simulink model "ex4_sim"  (R2015b)
settings: Solver=VariableStepAuto  StartTime=0.0  StopTime=simtime  RelTol=1e-3
values from neighbouring files (symbols this model uses):
  enable_karnop = 1    [ex1.m]    (also in ex2.m = 0; ex3.m; ex4.m = 0; exall.m = 0)
  enable_sin = 1    [ex1.m]    (also in ex2.m = 0; ex3.m; ex4.m = 0; exall.m = 0)
  F_c = 0.001    [ex1.m]    (also in ex2.m; ex3.m; ex4.m; exall.m)
  J = (J1 + J2)    (= 3.6e-05)    [ex1.m]    (also in ex2.m; ex3.m; ex4.m)
  motor = motor_pars    [ex1.m]    (also in ex2.m; ex3.m; ex4.m)
  motor_L = motor_pars    [ex1.m]    (also in ex2.m; ex3.m; ex4.m)
  n = 5    [ex1.m]    (also in ex2.m; ex3.m; ex4.m; ex5.m)
  sim_step_v = 2.38    [ex1.m]    (also in ex2.m = 1; ex3.m; ex4.m = 10)
undefined symbols (not defined in the file or in its folder): T_fric
libraries: simulink x2
settings Model: Creator=gabras  LastModifiedBy=Lamn
settings SolverCC: ZeroCrossAlgorithm=Adaptive
settings DataIOCC: SaveFormat=Array
settings DebuggingCC: SolverPrmCheckMsg=warning
settings HardwareCC: ProdBitPerPointer=32  ProdLargestAtomicFloat=None  ProdIntDivRoundTo=Undefined  ProdEndianess=Unspecified  ProdWordSize=32  ProdHWDeviceType=32-bit Generic
settings GRTTargetCC: GeneratePreprocessorConditionals=Disable all
settings ConfigComp: CovModelRefEnable=Off  CovSFcnEnable=off

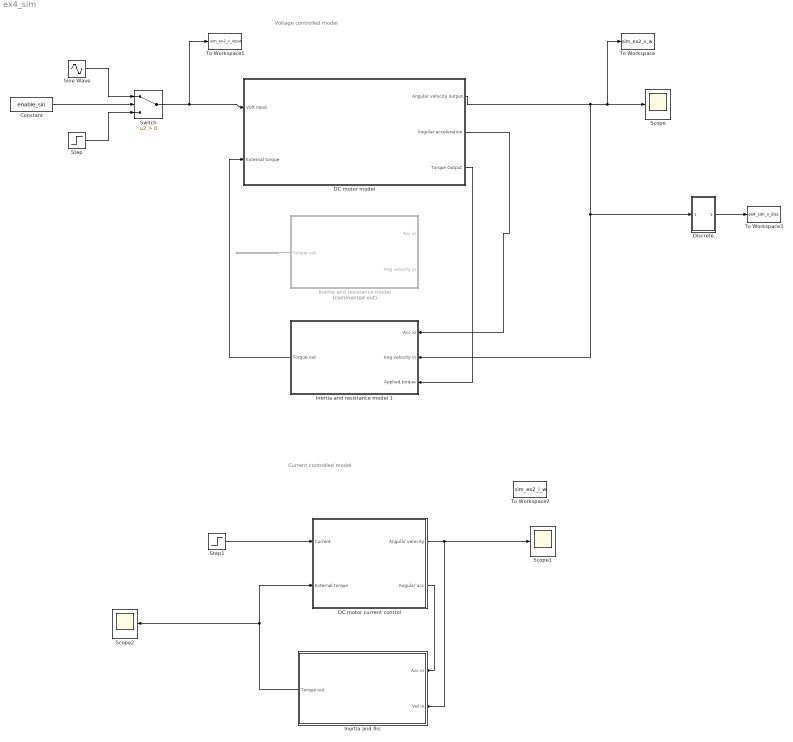
== system ex4_sim ==
  note: Current controlled model
  note: Voltage controlled model
  Constant : Constant  Value=enable_sin
  "DC motor current control " : Subsystem
  DC motor model : Subsystem
  Discrete : Subsystem
  Inertia and firc : Subsystem
  "Inertia and resistance model " : Subsystem  Commented=on
  Inertia and resistance model 1 : Subsystem
  Scope : Scope
  Scope1 : Scope
  Scope2 : Scope
  Sine Wave : Sin  SampleTime=0
  Step : Step  Time=0  After=sim_step_v  SampleTime=0
  Step1 : Step  Time=0  SampleTime=0
  Switch : Switch  Criteria=u2 > Threshold
  To Workspace : ToWorkspace  VariableName=sim_ex2_v_w  SaveFormat=Timeseries  SampleTime=-1
  To Workspace1 : ToWorkspace  VariableName=sim_ex2_v_input  SaveFormat=Timeseries  SampleTime=-1
  To Workspace2 : ToWorkspace  VariableName=sim_ex2_i_w  SaveFormat=Timeseries  SampleTime=-1
  To Workspace3 : ToWorkspace  VariableName=ex4_sim_v_disc  SaveFormat=Timeseries  SampleTime=-1
  wires:
  "Inertia and resistance model "/1(Torque out) -> ?
  DC motor model/2("Angular acceleration ") -> Inertia and resistance model 1/1(Acc in)
  Step1/1 -> "DC motor current control "/1(Current)
  "DC motor current control "/1(Angular velocity) -> Scope1/1, Inertia and firc/2(Vel in)
  "DC motor current control "/2(Angular acc) -> Inertia and firc/1(Acc in)
  Inertia and firc/1(Torque out) -> Scope2/1, "DC motor current control "/2(External torque)
  Step/1 -> Switch/3
  Sine Wave/1 -> Switch/1
  Switch/1 -> To Workspace1/1, DC motor model/1("Volt input ")
  Constant/1 -> Switch/2
  Inertia and resistance model 1/1(Torque out) -> DC motor model/2(External torque)
  DC motor model/3(Torque Output) -> Inertia and resistance model 1/3(Applied torque)
  DC motor model/1("Angular velocity output ") -> Discrete/1(In1), Inertia and resistance model 1/2(Ang velocity in), To Workspace/1, Scope/1
  Discrete/1(Out1) -> To Workspace3/1

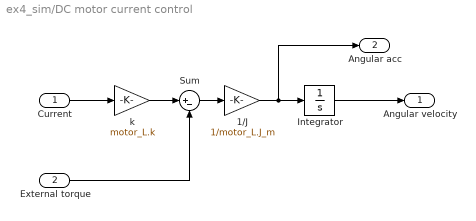
== system ex4_sim/DC motor current control  ==
  Current : Inport
  External torque : Inport  Port=2
  1/J : Gain  Gain=1/motor_L.J_m
  Integrator : Integrator
  Sum : Sum  Inputs=|+-
  "k " : Gain  Gain=motor_L.k
  Angular velocity : Outport
  Angular acc : Outport  Port=2
  wires:
  Current/1 -> "k "/1
  External torque/1 -> Sum/2
  "k "/1 -> Sum/1
  Sum/1 -> 1/J/1
  1/J/1 -> Angular acc/1, Integrator/1
  Integrator/1 -> Angular velocity/1

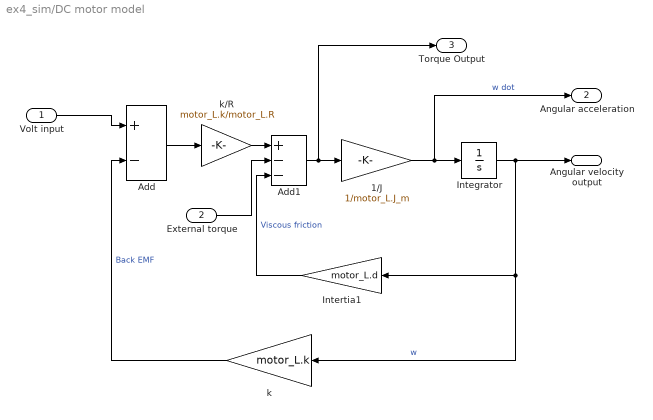
== system ex4_sim/DC motor model ==
  "Volt input " : Inport
  External torque : Inport  Port=2
  1/J : Gain  Gain=1/motor_L.J_m
  Add : Sum  Inputs=+-
  Add1 : Sum  Inputs=+--
  Integrator : Integrator
  Intertia1 : Gain  Gain=motor_L.d
  k : Gain  Gain=motor_L.k
  "k/R " : Gain  Gain=motor_L.k/motor_L.R
  "Angular velocity output " : Outport
  "Angular acceleration " : Outport  Port=2
  Torque Output : Outport  Port=3
  wires:
  "Volt input "/1 -> Add/1
  k/1 -> Add/2  "Back EMF"
  Add/1 -> "k/R "/1
  "k/R "/1 -> Add1/1
  Add1/1 -> Torque Output/1, 1/J/1
  1/J/1 -> "Angular acceleration "/1, Integrator/1  "w dot"
  Integrator/1 -> "Angular velocity output "/1, k/1, Intertia1/1  "w"
  External torque/1 -> Add1/2
  Intertia1/1 -> Add1/3  "Viscous friction"

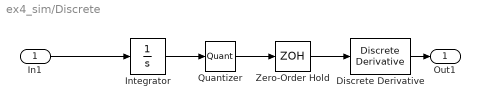
== system ex4_sim/Discrete ==
  In1 : Inport
  Discrete Derivative : simulink/Discrete/Discrete Derivative  gainval=1.0  ICPrevScaledInput=0.0  InputProcessing=Inherited  OutMin=[]  OutMax=[]  OutDataType=fixdt(1, 16)  OutScaling=2^-10  DoSatur=off
  Integrator : Integrator
  Quantizer : Quantizer  QuantizationInterval=sim_quantization_interval
  Zero-Order Hold : ZeroOrderHold  SampleTime=1e-3
  Out1 : Outport
  wires:
  Quantizer/1 -> Zero-Order Hold/1
  Zero-Order Hold/1 -> Discrete Derivative/1
  Integrator/1 -> Quantizer/1
  In1/1 -> Integrator/1
  Discrete Derivative/1 -> Out1/1

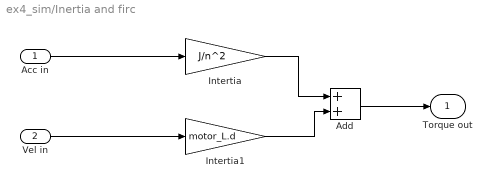
== system ex4_sim/Inertia and firc ==
  Acc in : Inport
  Vel in : Inport  Port=2
  Add : Sum
  Intertia : Gain  Gain=J/n^2
  Intertia1 : Gain  Gain=motor_L.d
  Torque out : Outport
  wires:
  Acc in/1 -> Intertia/1
  Vel in/1 -> Intertia1/1
  Intertia/1 -> Add/1
  Intertia1/1 -> Add/2
  Add/1 -> Torque out/1

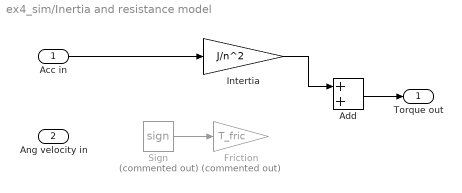
== system ex4_sim/Inertia and resistance model  ==
  Acc in : Inport
  Ang velocity in : Inport  Port=2
  Add : Sum
  Friction : Gain  Commented=on  Gain=T_fric
  Intertia : Gain  Gain=J/n^2
  Sign : Signum  Commented=on
  Torque out : Outport
  wires:
  Acc in/1 -> Intertia/1
  Sign/1 -> Friction/1
  Add/1 -> Torque out/1
  Intertia/1 -> Add/1

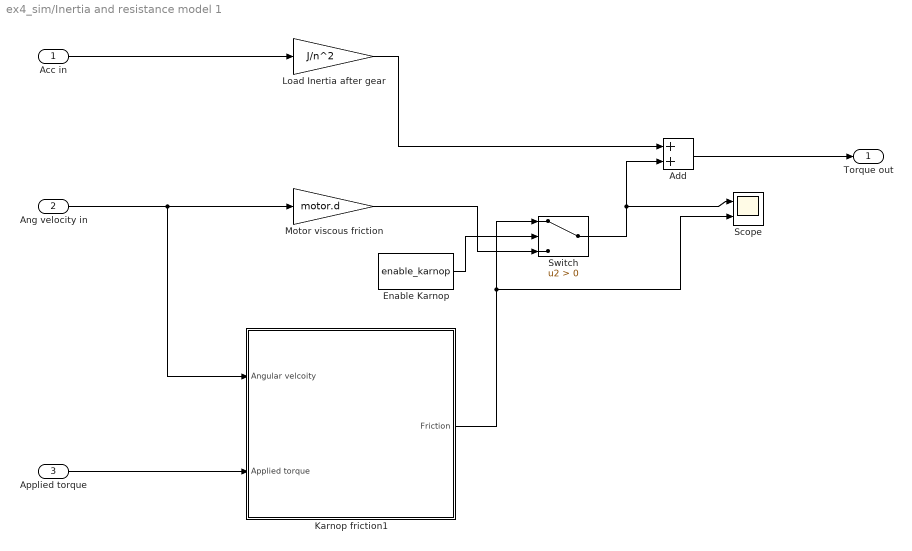
== system ex4_sim/Inertia and resistance model 1 ==
  Acc in : Inport
  Ang velocity in : Inport  Port=2
  Applied torque : Inport  Port=3
  Add : Sum
  Enable Karnop : Constant  Value=enable_karnop
  Karnop friction1 : Subsystem
  Load Inertia after gear : Gain  Gain=J/n^2
  Motor viscous friction : Gain  Gain=motor.d
  Scope : Scope  NumInputPorts=2
  Switch : Switch  Criteria=u2 > Threshold
  Torque out : Outport
  wires:
  Acc in/1 -> Load Inertia after gear/1
  Add/1 -> Torque out/1
  Load Inertia after gear/1 -> Add/1
  Ang velocity in/1 -> Karnop friction1/1(Angular velcoity), Motor viscous friction/1
  Motor viscous friction/1 -> Switch/3
  Karnop friction1/1(Friction) -> Switch/1, Scope/2
  Switch/1 -> Add/2, Scope/1
  Enable Karnop/1 -> Switch/2
  Applied torque/1 -> Karnop friction1/2("Applied torque ")

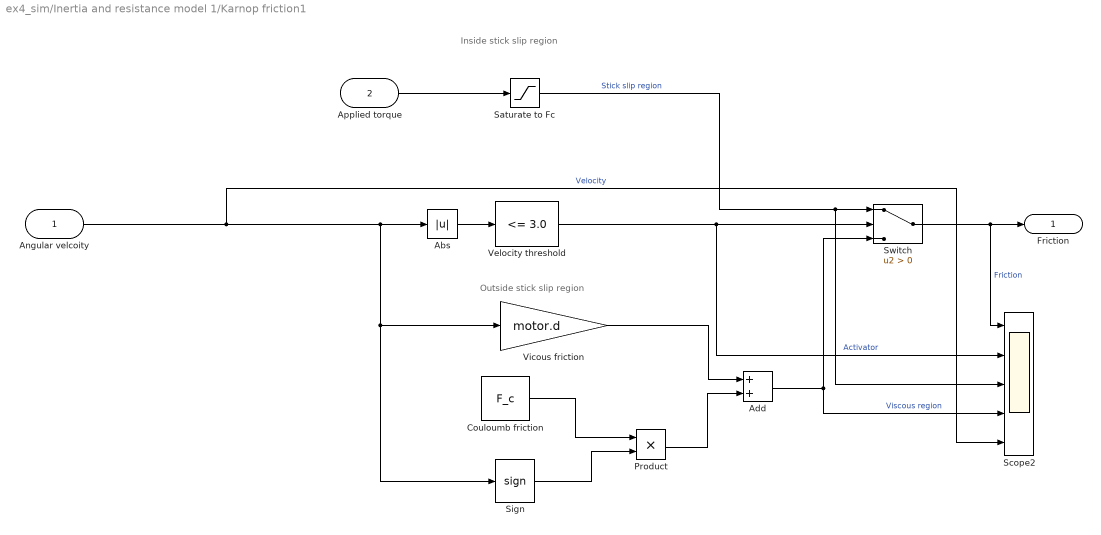
== system ex4_sim/Inertia and resistance model 1/Karnop friction1 ==
  note: Inside stick slip region
  note: Outside stick slip region
  Angular velcoity : Inport
  "Applied torque " : Inport  Port=2
  Abs : Abs
  Add : Sum
  Couloumb friction : Constant  Value=F_c
  Product : Product
  Saturate to Fc : Saturate  UpperLimit=F_c  LowerLimit=-F_c
  Scope2 : Scope  NumInputPorts=5
  Sign : Signum
  Switch : Switch  Criteria=u2 > Threshold
  "Velocity threshold " : simulink/Logic and Bit Operations/Compare To Constant  relop=<=  const=3.0  OutDataTypeStr=boolean  ZeroCross=off
  Vicous friction : Gain  Gain=motor.d
  Friction : Outport
  wires:
  Saturate to Fc/1 -> Scope2/3, Switch/1  "Stick slip region"
  Switch/1 -> Scope2/1, Friction/1  "Friction"
  Angular velcoity/1 -> Scope2/5, Abs/1, Vicous friction/1, Sign/1  "Velocity"
  "Velocity threshold "/1 -> Scope2/2, Switch/2  "Activator"
  Abs/1 -> "Velocity threshold "/1
  Product/1 -> Add/2
  Vicous friction/1 -> Add/1
  Couloumb friction/1 -> Product/1
  Sign/1 -> Product/2
  "Applied torque "/1 -> Saturate to Fc/1
  Add/1 -> Switch/3, Scope2/4  "Viscous region"
